simulink model "artemiscycles"  (R2016a)
settings: Solver=FixedStepAuto  StartTime=0.0  StopTime=3000  FixedStep=1  MaxStep=1e-1  RelTol=1e-3
values from neighbouring files (symbols this model uses):
  A = 2.25    [170315_artemis_w_others.mat]    (also in 170320_pulse_w_others.mat)
  cd = 0.3    [170315_artemis_w_others.mat]    (also in 170320_pulse_w_others.mat)
  cr = 0.01    [170315_artemis_w_others.mat]    (also in 170320_pulse_w_others.mat)
  eta = 0.8    [170315_artemis_w_others.mat]    (also in 170320_pulse_w_others.mat)
  g = 9.81    [170315_artemis_w_others.mat]    (also in 170320_pulse_w_others.mat)
  m = 1400    [170315_artemis_w_others.mat]    (also in 170320_pulse_w_others.mat)
  rho = 1.29    [170315_artemis_w_others.mat]    (also in 170320_pulse_w_others.mat)
libraries: drivecyclelib x1
settings Model: Creator=sebastian  LastModifiedBy=sebastian

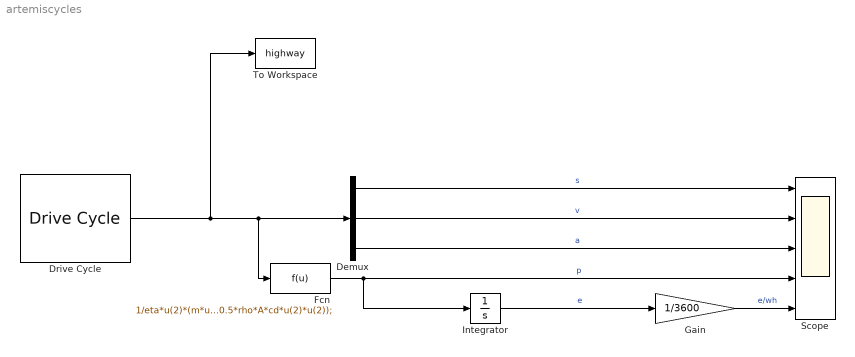
== system artemiscycles ==
  Demux : Demux  Outputs=3
  Drive Cycle : drivecyclelib/Drive Cycle  CycleName=ArtUrban  CycleRepeatsForever=off
  Fcn : Fcn  Expr=1/eta*u(2)*(m*u(3) + m*g*cr + 0.5*rho*A*cd*u(2)*u(2));
  Gain : Gain  Gain=1/3600
  Integrator : Integrator
  Scope : Scope  NumInputPorts=5
  To Workspace : ToWorkspace  VariableName=highway  SampleTime=-1
  wires:
  Demux/1 -> Scope/1  "s"
  Demux/2 -> Scope/2  "v"
  Demux/3 -> Scope/3  "a"
  Drive Cycle/1 -> To Workspace/1, Fcn/1, Demux/1
  Fcn/1 -> Scope/4, Integrator/1  "p"
  Integrator/1 -> Gain/1  "e"
  Gain/1 -> Scope/5  "e/wh"
